simulink library "testLib"  (R2024b)
settings: Solver=VariableStepAuto  StartTime=0.0  StopTime=10.0  RelTol=1e-3
libraries: simulink x3
settings Model: Creator=AK123700  LastModifiedBy=AK123700

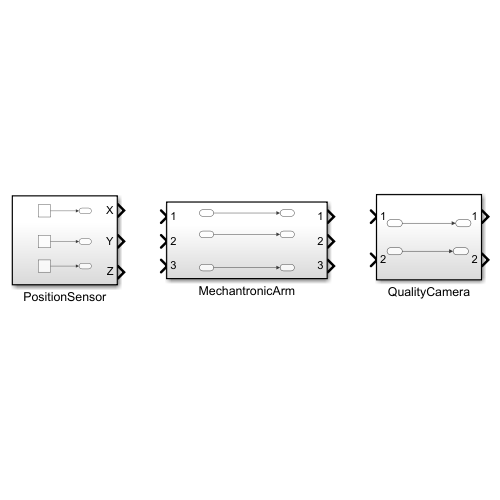
[thumbnail: Simulink's stored preview of the top-level diagram]
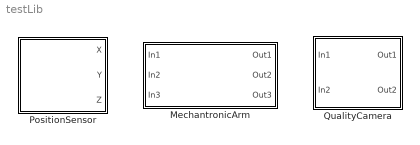
== system testLib ==
  MechantronicArm : Subsystem
  PositionSensor : Subsystem
  QualityCamera : Subsystem

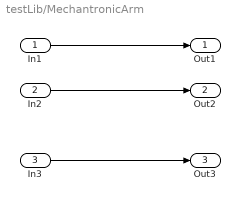
== system testLib/MechantronicArm ==
  In1 : Inport  OutDataTypeStr=uint8
  In2 : Inport  Port=2  OutDataTypeStr=uint8
  In3 : Inport  Port=3  OutDataTypeStr=uint8
  Out1 : Outport
  Out2 : Outport  Port=2
  Out3 : Outport  Port=3
  wires:
  In1/1 -> Out1/1
  In2/1 -> Out2/1
  In3/1 -> Out3/1

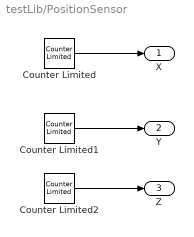
== system testLib/PositionSensor ==
  Counter Limited : simulink/Sources/Counter Limited  uplimit=7  tsamp=-1
  Counter Limited1 : simulink/Sources/Counter Limited  uplimit=8  tsamp=-1
  Counter Limited2 : simulink/Sources/Counter Limited  uplimit=8  tsamp=-1
  X : Outport  OutDataTypeStr=uint8
  Y : Outport  Port=2  OutDataTypeStr=uint8
  Z : Outport  Port=3  OutDataTypeStr=uint8
  wires:
  Counter Limited/1 -> X/1
  Counter Limited1/1 -> Y/1
  Counter Limited2/1 -> Z/1

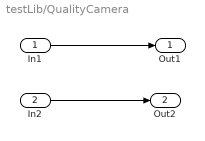
== system testLib/QualityCamera ==
  In1 : Inport  OutDataTypeStr=uint8
  In2 : Inport  Port=2  OutDataTypeStr=uint8
  Out1 : Outport
  Out2 : Outport  Port=2
  wires:
  In1/1 -> Out1/1
  In2/1 -> Out2/1
